simulink model "h_bridge_cascaded_five_level_inverter"  (R2022b)
settings: Solver=ode3  StartTime=0.0  StopTime=0.045  FixedStep=1e-6  RelTol=1e-3  EnableMultiTasking=on
undefined symbols (not defined in the file): fc, fr, Ma, ph
libraries: spsIGBTDiodeLib x328, simulink x164, spsDCVoltageSourceLib x82, spsCurrentMeasurementLib x41, spsSeriesRLCBranchLib x41, spsVoltageMeasurementLib x41, spspowerguiLib x1
(part 1 of 3)
settings Model: Creator=sruthi  LastModifiedBy=neotod
settings SolverCC: AlgebraicLoopSolver=TrustRegion  AutoInsertRateTranBlk=on
settings DataIOCC: LimitDataPoints=on  SaveFormat=Array  SignalLoggingSaveFormat=ModelDataLogs  ReturnWorkspaceOutputs=off
settings OptimizationCC: ExpressionDepthLimit=2147483647  LifeSpan=inf
settings DebuggingCC: UnderspecifiedInitializationDetection=Classic  MergeDetectMultiDrivingBlocksExec=none  SolverPrmCheckMsg=warning  FcnCallInpInsideContextMsg=warning  UnconnectedInputMsg=warning  UnconnectedOutputMsg=warning  UnconnectedLineMsg=warning  StateNameClashWarn=warning  SFUnexpectedBacktrackingDiag=warning  SFNoUnconditionalDefaultTransitionDiag=warning  SFExecutionAtInitializationDiag=none  SFMachineParentedDataDiag=warning  ArithmeticOperatorsInVariantConditions=warning
settings HardwareCC: ProdBitPerPointer=32  ProdBitPerSizeT=32  ProdBitPerPtrDiffT=32  ProdLargestAtomicFloat=None  ProdIntDivRoundTo=Undefined  ProdEndianess=Unspecified  ProdWordSize=32  ProdHWDeviceType=32-bit Generic
settings ModelReferenceCC: PropagateSignalLabelsOutOfModel=off
settings SFSimCC: SimUseLocalCustomCode=off  CustomCodeUndefinedFunction=UseInterfaceOnly
settings RTWCC: RTWUseLocalCustomCode=off
settings CodeAppCC: StateflowObjectComments=on
settings GRTTargetCC: TargetLangStandard=C89/C90 (ANSI)  CombineOutputUpdateFcns=off  GRTInterface=on
settings ConfigComp: CovMetricSettings=dw  CovSaveCumulativeToWorkspaceVar=on  CovSaveSingleToWorkspaceVar=on  CovExternalEMLEnable=off

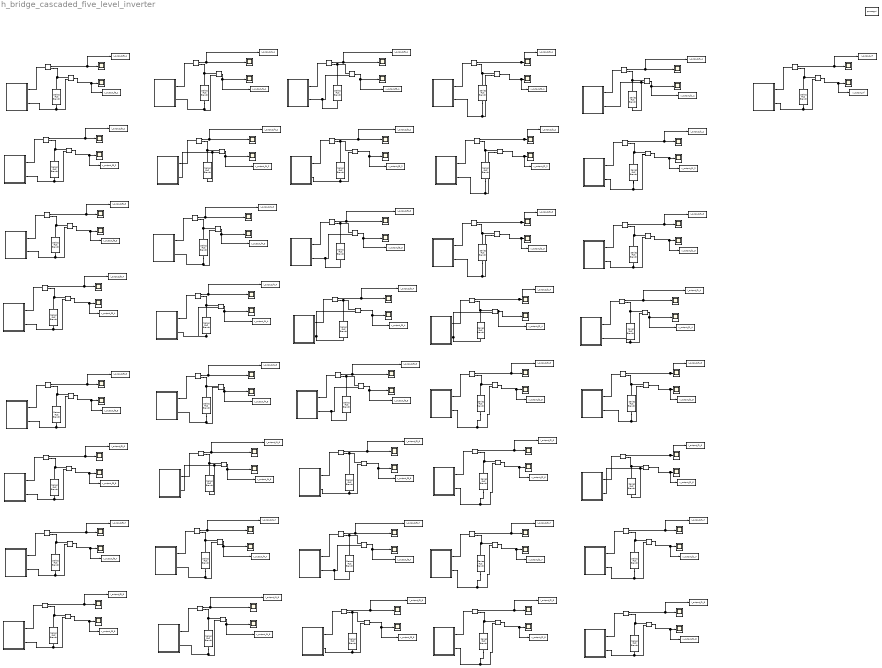
== system h_bridge_cascaded_five_level_inverter ==
  note: i_output_f6_5
  note: i_output_f3_6
  note: sim( '/path_to_simulinkmodel.slx' )
  note: currents
  note: voltages
  note: currents
  note: voltages
  note: currents
  note: voltages
  note: currents
  note: voltages
  note: CE short
  note: no fault
  note: collector open circuit
  note: gate signal removal
  note: voltages
  note: currents
  note: voltages
  note: currents
  note: voltages
  note: currents
  note: voltages
  note: voltages
  note: currents
  note: currents
  note: voltages
  note: voltages
  note: currents
  note: currents
  note: currents
  note: voltages
  note: emitter open circuit
  note: voltages
  note: currents
  note: currents
  note: voltages
  note: voltages
  note: currents
  note: voltages
  note: voltages
  note: currents
  note: currents
  note: currents
  note: voltages
  note: currents
  note: voltages
  note: voltages
  note: currents
  note: voltages
  note: currents
  note: voltages
  note: currents
  note: voltages
  note: currents
  note: voltages
  note: voltages
  note: currents
  note: voltages
  note: currents
  note: currents
  note: voltages
  note: currents
  note: voltages
  note: currents
  note: voltages
  note: currents
  note: currents
  note: voltages
  note: voltages
  note: voltages
  note: currents
  note: voltages
  note: currents
  note: currents
  note: voltages
  note: currents
  note: loose connection
  note: voltages
  note: currents
  note: voltages
  note: currents
  note: currents
  note: voltages
  note: voltages
  note: currents
  note: currents
  note: voltages
  note: voltages
  note: currents
  note: currents
  note: voltages
  Current Measurement{,1..3,5..34,42..48} (41 alike) : spsCurrentMeasurementLib/Current Measurement  PhasorSimulation=off  OutputType=Complex  PSBequivalent=0
  Phase A : Subsystem
  Phase A1 : Subsystem
  Phase A10 : Subsystem
  Phase A11 : Subsystem
  Phase A12 : Subsystem
  Phase A13 : Subsystem
  Phase A14 : Subsystem
  Phase A15 : Subsystem
  Phase A16 : Subsystem
  Phase A17 : Subsystem
  Phase A18 : Subsystem
  Phase A19 : Subsystem
  Phase A2 : Subsystem
  Phase A20 : Subsystem
  Phase A21 : Subsystem
  Phase A22 : Subsystem
  Phase A23 : Subsystem
  Phase A24 : Subsystem
  Phase A25 : Subsystem
  Phase A26 : Subsystem
  Phase A27 : Subsystem
  Phase A28 : Subsystem
  Phase A29 : Subsystem
  Phase A3 : Subsystem
  Phase A30 : Subsystem
  Phase A31 : Subsystem
  Phase A32 : Subsystem
  Phase A33 : Subsystem
  Phase A34 : Subsystem
  Phase A42 : Subsystem
  Phase A43 : Subsystem
  Phase A44 : Subsystem
  Phase A45 : Subsystem
  Phase A46 : Subsystem
  Phase A47 : Subsystem
  Phase A48 : Subsystem
  Phase A5 : Subsystem
  Phase A6 : Subsystem
  Phase A7 : Subsystem
  Phase A8 : Subsystem
  Phase A9 : Subsystem
  Scope{1..4,6..35,43..49} (41 alike) : Scope
  Series RLC Branch{,1..3,5..34,42..48} (41 alike) : spsSeriesRLCBranchLib/Series RLC Branch  LConnTagsString=__new0  RConnTagsString=__new0  BranchType=RL  Resistance=5  Inductance=5e-3  SetiL0=off  InitialCurrent=0  Capacitance=1e-6  Setx0=off  InitialVoltage=0  Measurements=None
  To Workspace : ToWorkspace  VariableName=v_output_nf  SaveFormat=Timeseries  SampleTime=-1
  To Workspace1 : ToWorkspace  VariableName=v_output_f1_1  SaveFormat=Timeseries  SampleTime=-1
  To Workspace10 : ToWorkspace  VariableName=v_output_f4_1  SaveFormat=Timeseries  SampleTime=-1
  To Workspace11 : ToWorkspace  VariableName=i_output_f4_1  SaveFormat=Timeseries  SampleTime=-1
  To Workspace12 : ToWorkspace  VariableName=v_output_f5_1  SaveFormat=Timeseries  SampleTime=-1
  To Workspace13 : ToWorkspace  VariableName=i_output_f5_1  SaveFormat=Timeseries  SampleTime=-1
  To Workspace14 : ToWorkspace  VariableName=v_output_f1_2  SaveFormat=Timeseries  SampleTime=-1
  To Workspace15 : ToWorkspace  VariableName=i_output_f1_2  SaveFormat=Timeseries  SampleTime=-1
  To Workspace16 : ToWorkspace  VariableName=v_output_f1_3  SaveFormat=Timeseries  SampleTime=-1
  To Workspace17 : ToWorkspace  VariableName=i_output_f1_3  SaveFormat=Timeseries  SampleTime=-1
  To Workspace18 : ToWorkspace  VariableName=v_output_f1_4  SaveFormat=Timeseries  SampleTime=-1
  To Workspace19 : ToWorkspace  VariableName=v_output_f1_5  SaveFormat=Timeseries  SampleTime=-1
  To Workspace2 : ToWorkspace  VariableName=i_output_f1_1  SaveFormat=Timeseries  SampleTime=-1
  To Workspace20 : ToWorkspace  VariableName=i_output_f1_5  SaveFormat=Timeseries  SampleTime=-1
  To Workspace21 : ToWorkspace  VariableName=v_output_f1_6  SaveFormat=Timeseries  SampleTime=-1
  To Workspace22 : ToWorkspace  VariableName=i_output_f1_6  SaveFormat=Timeseries  SampleTime=-1
  To Workspace23 : ToWorkspace  VariableName=i_output_f1_4  SaveFormat=Timeseries  SampleTime=-1
  To Workspace24 : ToWorkspace  VariableName=v_output_f1_7  SaveFormat=Timeseries  SampleTime=-1
  To Workspace25 : ToWorkspace  VariableName=i_output_f1_7  SaveFormat=Timeseries  SampleTime=-1
  To Workspace26 : ToWorkspace  VariableName=v_output_f1_8  SaveFormat=Timeseries  SampleTime=-1
  To Workspace27 : ToWorkspace  VariableName=i_output_f1_8  SaveFormat=Timeseries  SampleTime=-1
  To Workspace28 : ToWorkspace  VariableName=v_output_f2_2  SaveFormat=Timeseries  SampleTime=-1
  To Workspace29 : ToWorkspace  VariableName=i_output_f2_2  SaveFormat=Timeseries  SampleTime=-1
  To Workspace3 : ToWorkspace  VariableName=i_output_nf  SaveFormat=Timeseries  SampleTime=-1
  To Workspace30 : ToWorkspace  VariableName=v_output_f2_4  SaveFormat=Timeseries  SampleTime=-1
  To Workspace31 : ToWorkspace  VariableName=i_output_f2_4  SaveFormat=Timeseries  SampleTime=-1
  To Workspace32 : ToWorkspace  VariableName=v_output_f2_3  SaveFormat=Timeseries  SampleTime=-1
  To Workspace33 : ToWorkspace  VariableName=i_output_f2_3  SaveFormat=Timeseries  SampleTime=-1
  To Workspace34 : ToWorkspace  VariableName=v_output_f2_6  SaveFormat=Timeseries  SampleTime=-1
  To Workspace35 : ToWorkspace  VariableName=i_output_f2_6  SaveFormat=Timeseries  SampleTime=-1
  To Workspace36 : ToWorkspace  VariableName=v_output_f2_8  SaveFormat=Timeseries  SampleTime=-1
  To Workspace37 : ToWorkspace  VariableName=i_output_f2_8  SaveFormat=Timeseries  SampleTime=-1
  To Workspace38 : ToWorkspace  VariableName=v_output_f2_7  SaveFormat=Timeseries  SampleTime=-1
  To Workspace39 : ToWorkspace  VariableName=i_output_f2_7  SaveFormat=Timeseries  SampleTime=-1
  To Workspace4 : ToWorkspace  VariableName=v_output_f2_1  SaveFormat=Timeseries  SampleTime=-1
  To Workspace40 : ToWorkspace  VariableName=v_output_f2_5  SaveFormat=Timeseries  SampleTime=-1
  To Workspace41 : ToWorkspace  VariableName=i_output_f2_5  SaveFormat=Timeseries  SampleTime=-1
  To Workspace42 : ToWorkspace  VariableName=v_output_f3_2  SaveFormat=Timeseries  SampleTime=-1
  To Workspace43 : ToWorkspace  VariableName=i_output_f3_2  SaveFormat=Timeseries  SampleTime=-1
  To Workspace44 : ToWorkspace  VariableName=v_output_f3_4  SaveFormat=Timeseries  SampleTime=-1
  To Workspace45 : ToWorkspace  VariableName=i_output_f3_4  SaveFormat=Timeseries  SampleTime=-1
  To Workspace46 : ToWorkspace  VariableName=v_output_f3_3  SaveFormat=Timeseries  SampleTime=-1
  To Workspace47 : ToWorkspace  VariableName=i_output_f3_3  SaveFormat=Timeseries  SampleTime=-1
  To Workspace48 : ToWorkspace  VariableName=v_output_f3_6  SaveFormat=Timeseries  SampleTime=-1
  To Workspace49 : ToWorkspace  VariableName=i_output_f3_6  SaveFormat=Timeseries  SampleTime=-1
  To Workspace5 : ToWorkspace  VariableName=i_output_f2_1  SaveFormat=Timeseries  SampleTime=-1
  To Workspace50 : ToWorkspace  VariableName=v_output_f3_8  SaveFormat=Timeseries  SampleTime=-1
  To Workspace51 : ToWorkspace  VariableName=i_output_f3_8  SaveFormat=Timeseries  SampleTime=-1
  To Workspace52 : ToWorkspace  VariableName=v_output_f3_7  SaveFormat=Timeseries  SampleTime=-1
  To Workspace53 : ToWorkspace  VariableName=i_output_f3_7  SaveFormat=Timeseries  SampleTime=-1
  To Workspace54 : ToWorkspace  VariableName=v_output_f3_5  SaveFormat=Timeseries  SampleTime=-1
  To Workspace55 : ToWorkspace  VariableName=i_output_f3_5  SaveFormat=Timeseries  SampleTime=-1
  To Workspace56 : ToWorkspace  VariableName=v_output_f4_2  SaveFormat=Timeseries  SampleTime=-1
  To Workspace57 : ToWorkspace  VariableName=i_output_f4_2  SaveFormat=Timeseries  SampleTime=-1
  To Workspace58 : ToWorkspace  VariableName=v_output_f4_3  SaveFormat=Timeseries  SampleTime=-1
  To Workspace59 : ToWorkspace  VariableName=i_output_f4_3  SaveFormat=Timeseries  SampleTime=-1
  To Workspace6 : ToWorkspace  VariableName=v_output_f3_1  SaveFormat=Timeseries  SampleTime=-1
  To Workspace60 : ToWorkspace  VariableName=v_output_f4_4  SaveFormat=Timeseries  SampleTime=-1
  To Workspace61 : ToWorkspace  VariableName=i_output_f4_4  SaveFormat=Timeseries  SampleTime=-1
  To Workspace62 : ToWorkspace  VariableName=v_output_f4_5  SaveFormat=Timeseries  SampleTime=-1
  To Workspace63 : ToWorkspace  VariableName=i_output_f4_5  SaveFormat=Timeseries  SampleTime=-1
  To Workspace64 : ToWorkspace  VariableName=v_output_f4_6  SaveFormat=Timeseries  SampleTime=-1
  To Workspace65 : ToWorkspace  VariableName=i_output_f4_6  SaveFormat=Timeseries  SampleTime=-1
  To Workspace66 : ToWorkspace  VariableName=v_output_f4_7  SaveFormat=Timeseries  SampleTime=-1
  To Workspace67 : ToWorkspace  VariableName=i_output_f4_7  SaveFormat=Timeseries  SampleTime=-1
  To Workspace68 : ToWorkspace  VariableName=v_output_f4_8  SaveFormat=Timeseries  SampleTime=-1
  To Workspace69 : ToWorkspace  VariableName=i_output_f4_8  SaveFormat=Timeseries  SampleTime=-1
  To Workspace7 : ToWorkspace  VariableName=i_output_f3_1  SaveFormat=Timeseries  SampleTime=-1
  To Workspace84 : ToWorkspace  VariableName=v_output_f5_2  SaveFormat=Timeseries  SampleTime=-1
  To Workspace85 : ToWorkspace  VariableName=i_output_f5_2  SaveFormat=Timeseries  SampleTime=-1
  To Workspace86 : ToWorkspace  VariableName=v_output_f5_3  SaveFormat=Timeseries  SampleTime=-1
  To Workspace87 : ToWorkspace  VariableName=i_output_f5_3  SaveFormat=Timeseries  SampleTime=-1
  To Workspace88 : ToWorkspace  VariableName=v_output_f5_4  SaveFormat=Timeseries  SampleTime=-1
  To Workspace89 : ToWorkspace  VariableName=i_output_f5_4  SaveFormat=Timeseries  SampleTime=-1
  To Workspace90 : ToWorkspace  VariableName=v_output_f5_5  SaveFormat=Timeseries  SampleTime=-1
  To Workspace91 : ToWorkspace  VariableName=i_output_f5_5  SaveFormat=Timeseries  SampleTime=-1
  To Workspace92 : ToWorkspace  VariableName=v_output_f5_6  SaveFormat=Timeseries  SampleTime=-1
  To Workspace93 : ToWorkspace  VariableName=i_output_f5_6  SaveFormat=Timeseries  SampleTime=-1
  To Workspace94 : ToWorkspace  VariableName=v_output_f5_7  SaveFormat=Timeseries  SampleTime=-1
  To Workspace95 : ToWorkspace  VariableName=i_output_f5_7  SaveFormat=Timeseries  SampleTime=-1
  To Workspace96 : ToWorkspace  VariableName=v_output_f5_8  SaveFormat=Timeseries  SampleTime=-1
  To Workspace97 : ToWorkspace  VariableName=i_output_f5_8  SaveFormat=Timeseries  SampleTime=-1
  Voltage Measurement{,1..3,5..34,42..48} (41 alike) : spsVoltageMeasurementLib/Voltage Measurement  PhasorSimulation=off  OutputType=Complex  PSBequivalent=0
  current{,1..3,5..34,42..48} (41 alike) : Scope
  powergui : spspowerguiLib/powergui  Priority=1  SimulationMode=Discrete  SampleTime=100e-6  frequency=60  Iterations=50  frequencyindice=0  Pbase=100e6  ErrMax=1e-4  UnitsV=kV  UnitsW=MW  buscounter=0  FunctionMessages=off  echomessages=off  EnableUseOfTLC=off  CurrentSourceSwitches=off  DisableSnubberDevices=off  DisableRonSwitches=off  DisableVfSwitches=off  DisplayEquations=off  AutomaticDiscreteSolvers=off  SolverType=Tustin/Backward Euler (TBE)  Interpol=off  ExternalGateDelay=off  methode=off  Ts=100  x0status=blocks  SPID=off  SwTol=0  HookPort=off  NonlinearTolerance=1e-4  nMaxIteration=100  ContinueOnMaxIteration=off  RestoreLinks=warning  ResistiveCurrentMeasurement=off  Frange=[0:2:500]  Ylog=off  Xlog=on  ShowGrid=off  save=off  variable=ZData  structure=ScopeData  ZoomFFT=on  StartTime=0.0  cycles=1  DisplayStyle=1  fundamental=60  FreqAxis=off  MaxFrequency=1000  frequencyindicesteady=1  RmsSteady=1  display=off
  wires:
  Voltage Measurement/1 -> To Workspace/1, Scope1/1
  Current Measurement/1 -> To Workspace3/1, current/1
  Current Measurement1/1 -> To Workspace2/1, current1/1
  Voltage Measurement1/1 -> To Workspace1/1, Scope2/1
  Voltage Measurement3/1 -> To Workspace6/1, Scope4/1
  Current Measurement3/1 -> To Workspace7/1, current3/1
  Current Measurement5/1 -> To Workspace11/1, current5/1
  Voltage Measurement5/1 -> To Workspace10/1, Scope6/1
  Current Measurement7/1 -> To Workspace15/1, current7/1
  Voltage Measurement7/1 -> To Workspace14/1, Scope8/1
  Voltage Measurement8/1 -> To Workspace16/1, Scope9/1
  Current Measurement8/1 -> To Workspace17/1, current8/1
  Voltage Measurement11/1 -> To Workspace21/1, Scope12/1
  Voltage Measurement10/1 -> To Workspace19/1, Scope11/1
  Current Measurement11/1 -> To Workspace22/1, current11/1
  Current Measurement9/1 -> To Workspace23/1, current9/1
  Voltage Measurement9/1 -> To Workspace18/1, Scope10/1
  Current Measurement10/1 -> To Workspace20/1, current10/1
  Current Measurement13/1 -> To Workspace27/1, current13/1
  Voltage Measurement12/1 -> To Workspace24/1, Scope13/1
  Voltage Measurement13/1 -> To Workspace26/1, Scope14/1
  Current Measurement12/1 -> To Workspace25/1, current12/1
  Voltage Measurement2/1 -> To Workspace4/1, Scope3/1
  Current Measurement2/1 -> To Workspace5/1, current2/1
  Current Measurement14/1 -> To Workspace29/1, current14/1
  Voltage Measurement14/1 -> To Workspace28/1, Scope15/1
  Current Measurement15/1 -> To Workspace31/1, current15/1
  Voltage Measurement15/1 -> To Workspace30/1, Scope16/1
  Current Measurement16/1 -> To Workspace33/1, current16/1
  Voltage Measurement16/1 -> To Workspace32/1, Scope17/1
  Current Measurement17/1 -> To Workspace35/1, current17/1
  Voltage Measurement17/1 -> To Workspace34/1, Scope18/1
  Voltage Measurement19/1 -> To Workspace38/1, Scope20/1
  Voltage Measurement18/1 -> To Workspace36/1, Scope19/1
  Current Measurement18/1 -> To Workspace37/1, current18/1
  Current Measurement19/1 -> To Workspace39/1, current19/1
  Current Measurement20/1 -> To Workspace41/1, current20/1
  Voltage Measurement20/1 -> To Workspace40/1, Scope21/1
  Current Measurement21/1 -> To Workspace43/1, current21/1
  Voltage Measurement21/1 -> To Workspace42/1, Scope22/1
  Voltage Measurement22/1 -> To Workspace44/1, Scope23/1
  Current Measurement22/1 -> To Workspace45/1, current22/1
  Current Measurement23/1 -> To Workspace47/1, current23/1
  Voltage Measurement23/1 -> To Workspace46/1, Scope24/1
  Voltage Measurement24/1 -> To Workspace48/1, Scope25/1
  Current Measurement24/1 -> To Workspace49/1, current24/1
  Voltage Measurement27/1 -> To Workspace54/1, Scope28/1
  Current Measurement26/1 -> To Workspace53/1, current26/1
  Voltage Measurement26/1 -> To Workspace52/1, Scope27/1
  Current Measurement25/1 -> To Workspace51/1, current25/1
  Current Measurement27/1 -> To Workspace55/1, current27/1
  Voltage Measurement25/1 -> To Workspace50/1, Scope26/1
  Current Measurement28/1 -> To Workspace57/1, current28/1
  Voltage Measurement28/1 -> To Workspace56/1, Scope29/1
  Voltage Measurement29/1 -> To Workspace60/1, Scope30/1
  Current Measurement29/1 -> To Workspace61/1, current29/1
  Current Measurement30/1 -> To Workspace59/1, current30/1
  Voltage Measurement30/1 -> To Workspace58/1, Scope31/1
  Current Measurement33/1 -> To Workspace67/1, current33/1
  Current Measurement32/1 -> To Workspace69/1, current32/1
  Voltage Measurement33/1 -> To Workspace66/1, Scope34/1
  Voltage Measurement32/1 -> To Workspace68/1, Scope33/1
  Voltage Measurement31/1 -> To Workspace64/1, Scope32/1
  Current Measurement31/1 -> To Workspace65/1, current31/1
  Current Measurement34/1 -> To Workspace63/1, current34/1
  Voltage Measurement34/1 -> To Workspace62/1, Scope35/1
  Voltage Measurement6/1 -> To Workspace12/1, Scope7/1
  Current Measurement6/1 -> To Workspace13/1, current6/1
  Current Measurement42/1 -> To Workspace85/1, current42/1
  Voltage Measurement42/1 -> To Workspace84/1, Scope43/1
  Current Measurement44/1 -> To Workspace87/1, current44/1
  Voltage Measurement44/1 -> To Workspace86/1, Scope45/1
  Current Measurement43/1 -> To Workspace89/1, current43/1
  Voltage Measurement43/1 -> To Workspace88/1, Scope44/1
  Voltage Measurement47/1 -> To Workspace94/1, Scope48/1
  Voltage Measurement46/1 -> To Workspace96/1, Scope47/1
  Current Measurement48/1 -> To Workspace91/1, current48/1
  Current Measurement47/1 -> To Workspace95/1, current47/1
  Voltage Measurement48/1 -> To Workspace90/1, Scope49/1
  Current Measurement45/1 -> To Workspace93/1, current45/1
  Current Measurement46/1 -> To Workspace97/1, current46/1
  Voltage Measurement45/1 -> To Workspace92/1, Scope46/1
  connections:
  Voltage Measurement/LConn1 -- Series RLC Branch/LConn1 -- Current Measurement/RConn1
  Phase A/RConn1 -- Current Measurement/LConn1
  Phase A/RConn2 -- Series RLC Branch/RConn1 -- Voltage Measurement/LConn2
  Current Measurement1/RConn1 -- Series RLC Branch1/LConn1 -- Voltage Measurement1/LConn1
  Series RLC Branch1/RConn1 -- Phase A1/RConn2 -- Voltage Measurement1/LConn2
  Phase A1/RConn1 -- Current Measurement1/LConn1
  Phase A3/RConn2 -- Voltage Measurement3/LConn2 -- Series RLC Branch3/RConn1
  Current Measurement3/RConn1 -- Series RLC Branch3/LConn1 -- Voltage Measurement3/LConn1
  Phase A3/RConn1 -- Current Measurement3/LConn1
  Current Measurement5/RConn1 -- Series RLC Branch5/LConn1 -- Voltage Measurement5/LConn1
  Series RLC Branch5/RConn1 -- Phase A5/RConn2 -- Voltage Measurement5/LConn2
  Phase A5/RConn1 -- Current Measurement5/LConn1
  Voltage Measurement7/LConn2 -- Phase A7/RConn2 -- Series RLC Branch7/RConn1
  Current Measurement7/RConn1 -- Series RLC Branch7/LConn1 -- Voltage Measurement7/LConn1
  Phase A7/RConn1 -- Current Measurement7/LConn1
  Current Measurement8/RConn1 -- Series RLC Branch8/LConn1 -- Voltage Measurement8/LConn1
  Voltage Measurement8/LConn2 -- Phase A8/RConn2 -- Series RLC Branch8/RConn1
  Phase A8/RConn1 -- Current Measurement8/LConn1
  Current Measurement11/RConn1 -- Voltage Measurement11/LConn1 -- Series RLC Branch11/LConn1
  Current Measurement10/RConn1 -- Voltage Measurement10/LConn1 -- Series RLC Branch10/LConn1
  Voltage Measurement10/LConn2 -- Phase A10/RConn2 -- Series RLC Branch10/RConn1
  Current Measurement9/RConn1 -- Series RLC Branch9/LConn1 -- Voltage Measurement9/LConn1
  Series RLC Branch9/RConn1 -- Voltage Measurement9/LConn2 -- Phase A9/RConn2
  Voltage Measurement11/LConn2 -- Phase A11/RConn2 -- Series RLC Branch11/RConn1
  Phase A10/RConn1 -- Current Measurement10/LConn1
  Phase A11/RConn1 -- Current Measurement11/LConn1
  Phase A9/RConn1 -- Current Measurement9/LConn1
  Voltage Measurement13/LConn2 -- Phase A13/RConn2 -- Series RLC Branch13/RConn1
  Current Measurement12/RConn1 -- Series RLC Branch12/LConn1 -- Voltage Measurement12/LConn1
  Current Measurement13/RConn1 -- Series RLC Branch13/LConn1 -- Voltage Measurement13/LConn1
  Voltage Measurement12/LConn2 -- Phase A12/RConn2 -- Series RLC Branch12/RConn1
  Phase A13/RConn1 -- Current Measurement13/LConn1
  Phase A12/RConn1 -- Current Measurement12/LConn1
  Voltage Measurement2/LConn2 -- Phase A2/RConn2 -- Series RLC Branch2/RConn1
  Current Measurement2/RConn1 -- Voltage Measurement2/LConn1 -- Series RLC Branch2/LConn1
  Phase A2/RConn1 -- Current Measurement2/LConn1
  Current Measurement14/RConn1 -- Voltage Measurement14/LConn1 -- Series RLC Branch14/LConn1
  Voltage Measurement14/LConn2 -- Phase A14/RConn2 -- Series RLC Branch14/RConn1
  Phase A14/RConn1 -- Current Measurement14/LConn1
  Phase A15/RConn2 -- Series RLC Branch15/RConn1 -- Voltage Measurement15/LConn2
  Current Measurement15/RConn1 -- Voltage Measurement15/LConn1 -- Series RLC Branch15/LConn1
  Current Measurement16/RConn1 -- Voltage Measurement16/LConn1 -- Series RLC Branch16/LConn1
  Voltage Measurement16/LConn2 -- Phase A16/RConn2 -- Series RLC Branch16/RConn1
  Phase A15/RConn1 -- Current Measurement15/LConn1
  Phase A16/RConn1 -- Current Measurement16/LConn1
  Current Measurement18/RConn1 -- Series RLC Branch18/LConn1 -- Voltage Measurement18/LConn1
  Current Measurement19/RConn1 -- Series RLC Branch19/LConn1 -- Voltage Measurement19/LConn1
  Voltage Measurement17/LConn2 -- Phase A17/RConn2 -- Series RLC Branch17/RConn1
  Voltage Measurement18/LConn2 -- Phase A18/RConn2 -- Series RLC Branch18/RConn1
  Current Measurement17/RConn1 -- Series RLC Branch17/LConn1 -- Voltage Measurement17/LConn1
  Current Measurement20/RConn1 -- Series RLC Branch20/LConn1 -- Voltage Measurement20/LConn1
  Voltage Measurement20/LConn2 -- Phase A20/RConn2 -- Series RLC Branch20/RConn1
  Voltage Measurement19/LConn2 -- Phase A19/RConn2 -- Series RLC Branch19/RConn1
  Phase A19/RConn1 -- Current Measurement19/LConn1
  Phase A20/RConn1 -- Current Measurement20/LConn1
  Phase A18/RConn1 -- Current Measurement18/LConn1
  Phase A17/RConn1 -- Current Measurement17/LConn1
  Phase A21/RConn2 -- Voltage Measurement21/LConn2 -- Series RLC Branch21/RConn1
  Voltage Measurement21/LConn1 -- Current Measurement21/RConn1 -- Series RLC Branch21/LConn1
  Phase A21/RConn1 -- Current Measurement21/LConn1
  Phase A22/RConn2 -- Voltage Measurement22/LConn2 -- Series RLC Branch22/RConn1
  Voltage Measurement22/LConn1 -- Current Measurement22/RConn1 -- Series RLC Branch22/LConn1
  Series RLC Branch23/RConn1 -- Phase A23/RConn2 -- Voltage Measurement23/LConn2
  Voltage Measurement23/LConn1 -- Current Measurement23/RConn1 -- Series RLC Branch23/LConn1
  Phase A22/RConn1 -- Current Measurement22/LConn1
  Phase A23/RConn1 -- Current Measurement23/LConn1
  Voltage Measurement25/LConn1 -- Current Measurement25/RConn1 -- Series RLC Branch25/LConn1
  Phase A25/RConn2 -- Voltage Measurement25/LConn2 -- Series RLC Branch25/RConn1
  Phase A24/RConn2 -- Voltage Measurement24/LConn2 -- Series RLC Branch24/RConn1
  Series RLC Branch26/RConn1 -- Phase A26/RConn2 -- Voltage Measurement26/LConn2
  Voltage Measurement24/LConn1 -- Current Measurement24/RConn1 -- Series RLC Branch24/LConn1
  Voltage Measurement26/LConn1 -- Current Measurement26/RConn1 -- Series RLC Branch26/LConn1
  Series RLC Branch27/RConn1 -- Phase A27/RConn2 -- Voltage Measurement27/LConn2
  Voltage Measurement27/LConn1 -- Current Measurement27/RConn1 -- Series RLC Branch27/LConn1
  Phase A27/RConn1 -- Current Measurement27/LConn1
  Phase A26/RConn1 -- Current Measurement26/LConn1
  Phase A25/RConn1 -- Current Measurement25/LConn1
  Phase A24/RConn1 -- Current Measurement24/LConn1
  Current Measurement28/RConn1 -- Series RLC Branch28/LConn1 -- Voltage Measurement28/LConn1
  Series RLC Branch28/RConn1 -- Voltage Measurement28/LConn2 -- Phase A28/RConn2
  Phase A28/RConn1 -- Current Measurement28/LConn1
  Series RLC Branch29/RConn1 -- Phase A29/RConn2 -- Voltage Measurement29/LConn2
  Current Measurement30/RConn1 -- Series RLC Branch30/LConn1 -- Voltage Measurement30/LConn1
  Current Measurement29/RConn1 -- Series RLC Branch29/LConn1 -- Voltage Measurement29/LConn1
  Series RLC Branch30/RConn1 -- Phase A30/RConn2 -- Voltage Measurement30/LConn2
  Phase A30/RConn1 -- Current Measurement30/LConn1
  Phase A29/RConn1 -- Current Measurement29/LConn1
  Current Measurement32/RConn1 -- Series RLC Branch32/LConn1 -- Voltage Measurement32/LConn1
  Series RLC Branch32/RConn1 -- Phase A32/RConn2 -- Voltage Measurement32/LConn2
  Series RLC Branch33/RConn1 -- Phase A33/RConn2 -- Voltage Measurement33/LConn2
  Current Measurement33/RConn1 -- Series RLC Branch33/LConn1 -- Voltage Measurement33/LConn1
  Phase A31/RConn2 -- Series RLC Branch31/RConn1 -- Voltage Measurement31/LConn2
  Current Measurement34/RConn1 -- Series RLC Branch34/LConn1 -- Voltage Measurement34/LConn1
  Current Measurement31/RConn1 -- Series RLC Branch31/LConn1 -- Voltage Measurement31/LConn1
  Series RLC Branch34/RConn1 -- Phase A34/RConn2 -- Voltage Measurement34/LConn2
  Phase A34/RConn1 -- Current Measurement34/LConn1
  Phase A31/RConn1 -- Current Measurement31/LConn1
  Phase A33/RConn1 -- Current Measurement33/LConn1
  Phase A32/RConn1 -- Current Measurement32/LConn1
  Current Measurement6/RConn1 -- Series RLC Branch6/LConn1 -- Voltage Measurement6/LConn1
  Voltage Measurement6/LConn2 -- Phase A6/RConn2 -- Series RLC Branch6/RConn1
  Phase A6/RConn1 -- Current Measurement6/LConn1
  Voltage Measurement42/LConn2 -- Phase A42/RConn2 -- Series RLC Branch42/RConn1
  Current Measurement42/RConn1 -- Series RLC Branch42/LConn1 -- Voltage Measurement42/LConn1
  Phase A42/RConn1 -- Current Measurement42/LConn1
  Voltage Measurement43/LConn2 -- Phase A43/RConn2 -- Series RLC Branch43/RConn1
  Current Measurement43/RConn1 -- Series RLC Branch43/LConn1 -- Voltage Measurement43/LConn1
  Voltage Measurement44/LConn2 -- Phase A44/RConn2 -- Series RLC Branch44/RConn1
  Current Measurement44/RConn1 -- Series RLC Branch44/LConn1 -- Voltage Measurement44/LConn1
  Phase A44/RConn1 -- Current Measurement44/LConn1
  Phase A43/RConn1 -- Current Measurement43/LConn1
  Voltage Measurement46/LConn2 -- Phase A46/RConn2 -- Series RLC Branch46/RConn1
  Voltage Measurement45/LConn2 -- Phase A45/RConn2 -- Series RLC Branch45/RConn1
  Current Measurement45/RConn1 -- Series RLC Branch45/LConn1 -- Voltage Measurement45/LConn1
  Voltage Measurement47/LConn2 -- Phase A47/RConn2 -- Series RLC Branch47/RConn1
  Current Measurement47/RConn1 -- Series RLC Branch47/LConn1 -- Voltage Measurement47/LConn1
  Voltage Measurement48/LConn2 -- Phase A48/RConn2 -- Series RLC Branch48/RConn1
  Current Measurement48/RConn1 -- Series RLC Branch48/LConn1 -- Voltage Measurement48/LConn1
  Current Measurement46/RConn1 -- Series RLC Branch46/LConn1 -- Voltage Measurement46/LConn1
  Phase A47/RConn1 -- Current Measurement47/LConn1
  Phase A46/RConn1 -- Current Measurement46/LConn1
  Phase A45/RConn1 -- Current Measurement45/LConn1
  Phase A48/RConn1 -- Current Measurement48/LConn1

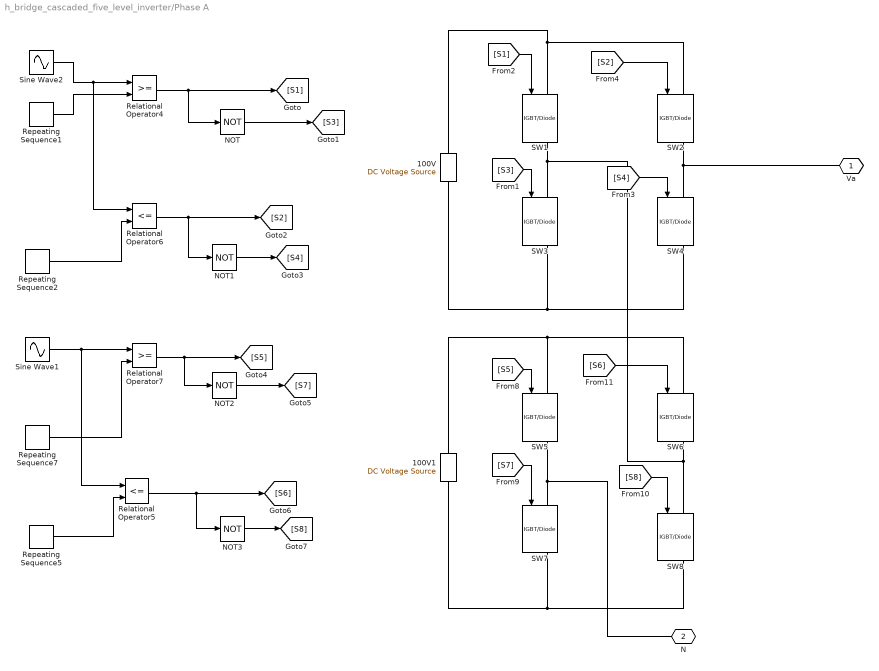
== system h_bridge_cascaded_five_level_inverter/Phase A ==
  100V : spsDCVoltageSourceLib/DC Voltage Source  Amplitude=100  Measurements=None
  100V1 : spsDCVoltageSourceLib/DC Voltage Source  Amplitude=100  Measurements=None
  NOT{,1..3} (4 alike) : Logic  Operator=NOT  AllPortsSameDT=off  OutDataTypeStr=boolean
  Relational Operator4 : RelationalOperator  OutDataTypeStr=boolean  InputSameDT=off
  Relational Operator5 : RelationalOperator  Operator=<=  OutDataTypeStr=boolean  InputSameDT=off
  Relational Operator6 : RelationalOperator  Operator=<=  OutDataTypeStr=boolean  InputSameDT=off
  Relational Operator7 : RelationalOperator  OutDataTypeStr=boolean  InputSameDT=off
  Repeating Sequence1 : simulink/Sources/Repeating Sequence  rep_seq_t=[0 0.00025 0.0005 0.00075 0.001]*(1/fr)*(1/fc)*(1/2)  rep_seq_y="[0 1 0 -1 0  ]"
  Repeating Sequence2 : simulink/Sources/Repeating Sequence  rep_seq_t=[0 0.00025 0.0005 0.00075 0.001]*(1/fr)*(1/fc)*(1/2)  rep_seq_y=[ 0 -1 0 1 0 ]
  Repeating Sequence5 : simulink/Sources/Repeating Sequence  rep_seq_t=[0 0.00025 0.0005 0.00075 0.001]*(1/fr)*(1/fc)*(1/2)  rep_seq_y=[1 0 -1 0 1]
  Repeating Sequence7 : simulink/Sources/Repeating Sequence  rep_seq_t=[0 0.00025 0.0005 0.00075 0.001]*(1/fr)*(1/fc)*(1/2)  rep_seq_y=[-1 0 1 0 -1]
  SW{1..8} (8 alike) : spsIGBTDiodeLib/IGBT//Diode  Ron=1e-3  Rs=1e5  Cs=inf  Measurements=on
  Sine Wave1 : Sin  Amplitude=Ma  Frequency=2*pi*fr  Phase=ph  SampleTime=0
  Sine Wave2 : Sin  Amplitude=Ma  Frequency=2*pi*fr  Phase=ph  SampleTime=0
  Va : PMIOPort  Tag=PMCPort  Side=Right
  N : PMIOPort  Tag=PMCPort  Port=2  Side=Right
  wires:
  Sine Wave2/1 -> Relational Operator4/1, Relational Operator6/1
  Repeating Sequence1/1 -> Relational Operator4/2
  Repeating Sequence2/1 -> Relational Operator6/2
  Relational Operator4/1 -> NOT/1, [S1]
  NOT/1 -> [S3]
  NOT1/1 -> [S4]
  Relational Operator6/1 -> [S2], NOT1/1
  Repeating Sequence7/1 -> Relational Operator7/2
  Repeating Sequence5/1 -> Relational Operator5/2
  Sine Wave1/1 -> Relational Operator7/1, Relational Operator5/1
  Relational Operator5/1 -> [S6], NOT3/1
  Relational Operator7/1 -> [S5], NOT2/1
  NOT2/1 -> [S7]
  NOT3/1 -> [S8]
  [S3] -> SW3/1
  [S4] -> SW4/1
  [S6] -> SW6/1
  [S5] -> SW5/1
  [S7] -> SW7/1
  [S8] -> SW8/1
  [S1] -> SW1/1
  [S2] -> SW2/1
  connections:
  Va/RConn1 -- SW2/RConn1 -- SW4/LConn1
  SW4/RConn1 -- 100V/LConn1 -- SW3/RConn1
  SW8/RConn1 -- 100V1/LConn1 -- SW7/RConn1
  SW1/RConn1 -- SW3/LConn1 -- SW6/RConn1 -- SW8/LConn1
  SW5/LConn1 -- 100V1/RConn1 -- SW6/LConn1
  N/RConn1 -- SW5/RConn1 -- SW7/LConn1
  100V/RConn1 -- SW2/LConn1 -- SW1/LConn1

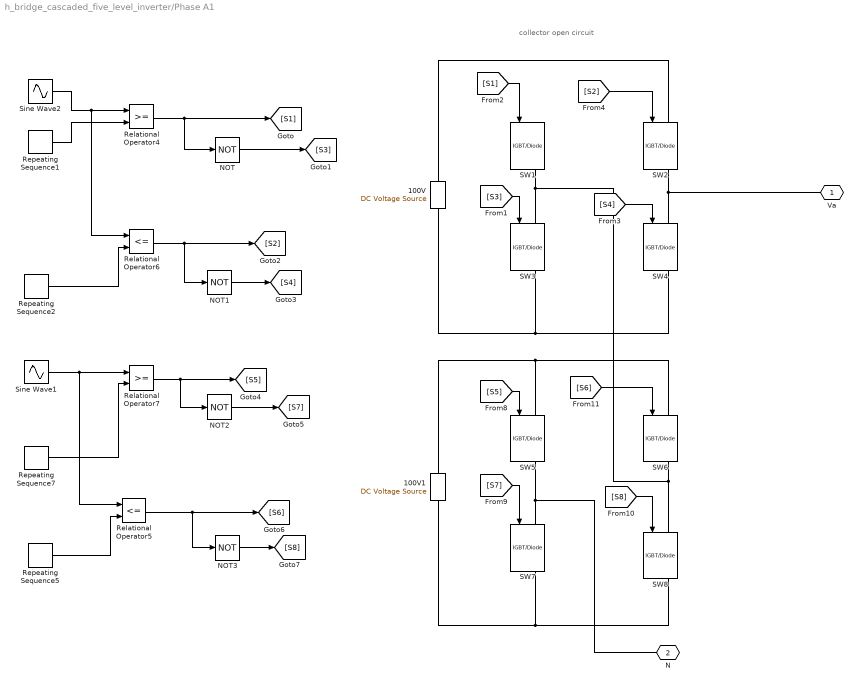
== system h_bridge_cascaded_five_level_inverter/Phase A1 ==
  note: collector open circuit
  100V : spsDCVoltageSourceLib/DC Voltage Source  Amplitude=100  Measurements=None
  100V1 : spsDCVoltageSourceLib/DC Voltage Source  Amplitude=100  Measurements=None
  NOT{,1..3} (4 alike) : Logic  Operator=NOT  AllPortsSameDT=off  OutDataTypeStr=boolean
  Relational Operator4 : RelationalOperator  OutDataTypeStr=boolean  InputSameDT=off
  Relational Operator5 : RelationalOperator  Operator=<=  OutDataTypeStr=boolean  InputSameDT=off
  Relational Operator6 : RelationalOperator  Operator=<=  OutDataTypeStr=boolean  InputSameDT=off
  Relational Operator7 : RelationalOperator  OutDataTypeStr=boolean  InputSameDT=off
  Repeating Sequence1 : simulink/Sources/Repeating Sequence  rep_seq_t=[0 0.00025 0.0005 0.00075 0.001]*(1/fr)*(1/fc)*(1/2)  rep_seq_y="[0 1 0 -1 0  ]"
  Repeating Sequence2 : simulink/Sources/Repeating Sequence  rep_seq_t=[0 0.00025 0.0005 0.00075 0.001]*(1/fr)*(1/fc)*(1/2)  rep_seq_y=[ 0 -1 0 1 0 ]
  Repeating Sequence5 : simulink/Sources/Repeating Sequence  rep_seq_t=[0 0.00025 0.0005 0.00075 0.001]*(1/fr)*(1/fc)*(1/2)  rep_seq_y=[1 0 -1 0 1]
  Repeating Sequence7 : simulink/Sources/Repeating Sequence  rep_seq_t=[0 0.00025 0.0005 0.00075 0.001]*(1/fr)*(1/fc)*(1/2)  rep_seq_y=[-1 0 1 0 -1]
  SW{1..8} (8 alike) : spsIGBTDiodeLib/IGBT//Diode  Ron=1e-3  Rs=1e5  Cs=inf  Measurements=on
  Sine Wave1 : Sin  Amplitude=Ma  Frequency=2*pi*fr  Phase=ph  SampleTime=0
  Sine Wave2 : Sin  Amplitude=Ma  Frequency=2*pi*fr  Phase=ph  SampleTime=0
  Va : PMIOPort  Tag=PMCPort  Side=Right
  N : PMIOPort  Tag=PMCPort  Port=2  Side=Right
  wires:
  Sine Wave2/1 -> Relational Operator4/1, Relational Operator6/1
  Repeating Sequence1/1 -> Relational Operator4/2
  Repeating Sequence2/1 -> Relational Operator6/2
  Relational Operator4/1 -> NOT/1, [S1]
  NOT/1 -> [S3]
  NOT1/1 -> [S4]
  Relational Operator6/1 -> [S2], NOT1/1
  Repeating Sequence7/1 -> Relational Operator7/2
  Repeating Sequence5/1 -> Relational Operator5/2
  Sine Wave1/1 -> Relational Operator7/1, Relational Operator5/1
  Relational Operator5/1 -> [S6], NOT3/1
  Relational Operator7/1 -> [S5], NOT2/1
  NOT2/1 -> [S7]
  NOT3/1 -> [S8]
  [S3] -> SW3/1
  [S4] -> SW4/1
  [S6] -> SW6/1
  [S5] -> SW5/1
  [S7] -> SW7/1
  [S8] -> SW8/1
  [S1] -> SW1/1
  [S2] -> SW2/1
  connections:
  Va/RConn1 -- SW2/RConn1 -- SW4/LConn1
  SW4/RConn1 -- 100V/LConn1 -- SW3/RConn1
  SW8/RConn1 -- 100V1/LConn1 -- SW7/RConn1
  SW1/RConn1 -- SW3/LConn1 -- SW6/RConn1 -- SW8/LConn1
  SW5/LConn1 -- 100V1/RConn1 -- SW6/LConn1
  N/RConn1 -- SW5/RConn1 -- SW7/LConn1
  SW2/LConn1 -- 100V/RConn1

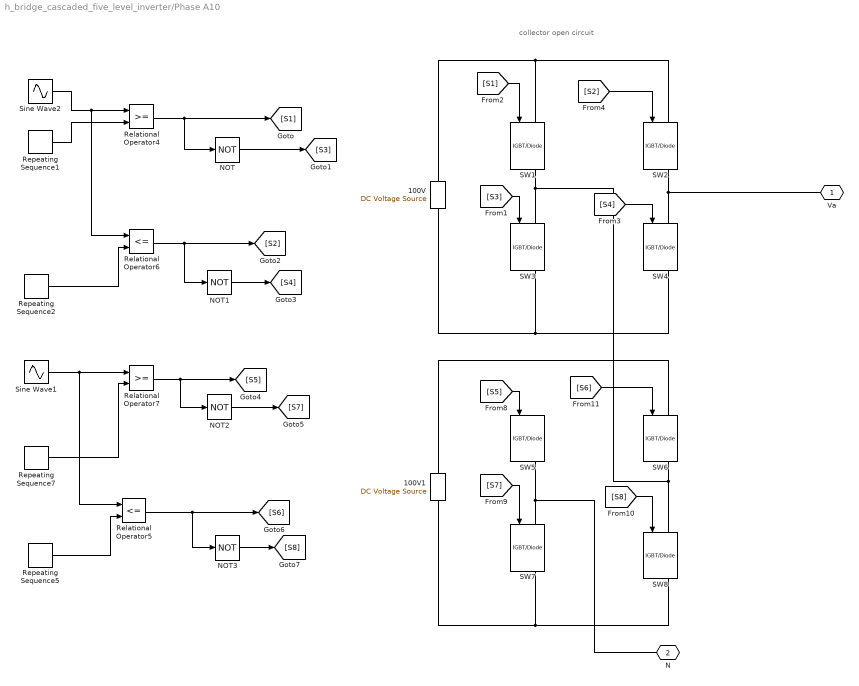
== system h_bridge_cascaded_five_level_inverter/Phase A10 ==
  note: collector open circuit
  100V : spsDCVoltageSourceLib/DC Voltage Source  Amplitude=100  Measurements=None
  100V1 : spsDCVoltageSourceLib/DC Voltage Source  Amplitude=100  Measurements=None
  NOT{,1..3} (4 alike) : Logic  Operator=NOT  AllPortsSameDT=off  OutDataTypeStr=boolean
  Relational Operator4 : RelationalOperator  OutDataTypeStr=boolean  InputSameDT=off
  Relational Operator5 : RelationalOperator  Operator=<=  OutDataTypeStr=boolean  InputSameDT=off
  Relational Operator6 : RelationalOperator  Operator=<=  OutDataTypeStr=boolean  InputSameDT=off
  Relational Operator7 : RelationalOperator  OutDataTypeStr=boolean  InputSameDT=off
  Repeating Sequence1 : simulink/Sources/Repeating Sequence  rep_seq_t=[0 0.00025 0.0005 0.00075 0.001]*(1/fr)*(1/fc)*(1/2)  rep_seq_y="[0 1 0 -1 0  ]"
  Repeating Sequence2 : simulink/Sources/Repeating Sequence  rep_seq_t=[0 0.00025 0.0005 0.00075 0.001]*(1/fr)*(1/fc)*(1/2)  rep_seq_y=[ 0 -1 0 1 0 ]
  Repeating Sequence5 : simulink/Sources/Repeating Sequence  rep_seq_t=[0 0.00025 0.0005 0.00075 0.001]*(1/fr)*(1/fc)*(1/2)  rep_seq_y=[1 0 -1 0 1]
  Repeating Sequence7 : simulink/Sources/Repeating Sequence  rep_seq_t=[0 0.00025 0.0005 0.00075 0.001]*(1/fr)*(1/fc)*(1/2)  rep_seq_y=[-1 0 1 0 -1]
  SW{1..8} (8 alike) : spsIGBTDiodeLib/IGBT//Diode  Ron=1e-3  Rs=1e5  Cs=inf  Measurements=on
  Sine Wave1 : Sin  Amplitude=Ma  Frequency=2*pi*fr  Phase=ph  SampleTime=0
  Sine Wave2 : Sin  Amplitude=Ma  Frequency=2*pi*fr  Phase=ph  SampleTime=0
  Va : PMIOPort  Tag=PMCPort  Side=Right
  N : PMIOPort  Tag=PMCPort  Port=2  Side=Right
  wires:
  Sine Wave2/1 -> Relational Operator4/1, Relational Operator6/1
  Repeating Sequence1/1 -> Relational Operator4/2
  Repeating Sequence2/1 -> Relational Operator6/2
  Relational Operator4/1 -> NOT/1, [S1]
  NOT/1 -> [S3]
  NOT1/1 -> [S4]
  Relational Operator6/1 -> [S2], NOT1/1
  Repeating Sequence7/1 -> Relational Operator7/2
  Repeating Sequence5/1 -> Relational Operator5/2
  Sine Wave1/1 -> Relational Operator7/1, Relational Operator5/1
  Relational Operator5/1 -> [S6], NOT3/1
  Relational Operator7/1 -> [S5], NOT2/1
  NOT2/1 -> [S7]
  NOT3/1 -> [S8]
  [S3] -> SW3/1
  [S4] -> SW4/1
  [S6] -> SW6/1
  [S5] -> SW5/1
  [S7] -> SW7/1
  [S8] -> SW8/1
  [S1] -> SW1/1
  [S2] -> SW2/1
  connections:
  Va/RConn1 -- SW2/RConn1 -- SW4/LConn1
  SW4/RConn1 -- 100V/LConn1 -- SW3/RConn1
  SW8/RConn1 -- 100V1/LConn1 -- SW7/RConn1
  SW1/RConn1 -- SW6/RConn1 -- SW8/LConn1 -- SW3/LConn1
  SW6/LConn1 -- 100V1/RConn1
  N/RConn1 -- SW5/RConn1 -- SW7/LConn1
  100V/RConn1 -- SW1/LConn1 -- SW2/LConn1

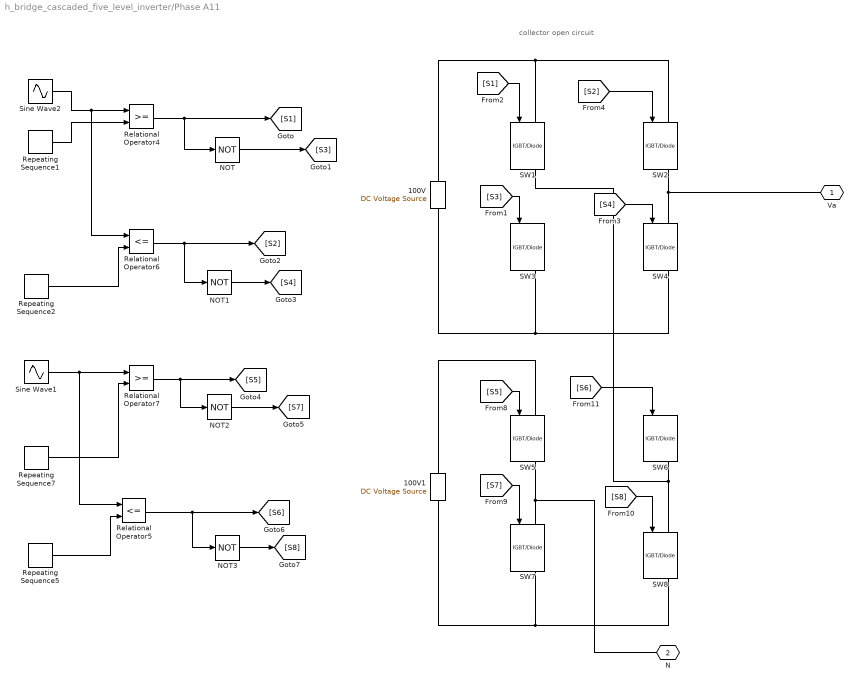
== system h_bridge_cascaded_five_level_inverter/Phase A11 ==
  note: collector open circuit
  100V : spsDCVoltageSourceLib/DC Voltage Source  Amplitude=100  Measurements=None
  100V1 : spsDCVoltageSourceLib/DC Voltage Source  Amplitude=100  Measurements=None
  NOT{,1..3} (4 alike) : Logic  Operator=NOT  AllPortsSameDT=off  OutDataTypeStr=boolean
  Relational Operator4 : RelationalOperator  OutDataTypeStr=boolean  InputSameDT=off
  Relational Operator5 : RelationalOperator  Operator=<=  OutDataTypeStr=boolean  InputSameDT=off
  Relational Operator6 : RelationalOperator  Operator=<=  OutDataTypeStr=boolean  InputSameDT=off
  Relational Operator7 : RelationalOperator  OutDataTypeStr=boolean  InputSameDT=off
  Repeating Sequence1 : simulink/Sources/Repeating Sequence  rep_seq_t=[0 0.00025 0.0005 0.00075 0.001]*(1/fr)*(1/fc)*(1/2)  rep_seq_y="[0 1 0 -1 0  ]"
  Repeating Sequence2 : simulink/Sources/Repeating Sequence  rep_seq_t=[0 0.00025 0.0005 0.00075 0.001]*(1/fr)*(1/fc)*(1/2)  rep_seq_y=[ 0 -1 0 1 0 ]
  Repeating Sequence5 : simulink/Sources/Repeating Sequence  rep_seq_t=[0 0.00025 0.0005 0.00075 0.001]*(1/fr)*(1/fc)*(1/2)  rep_seq_y=[1 0 -1 0 1]
  Repeating Sequence7 : simulink/Sources/Repeating Sequence  rep_seq_t=[0 0.00025 0.0005 0.00075 0.001]*(1/fr)*(1/fc)*(1/2)  rep_seq_y=[-1 0 1 0 -1]
  SW{1..8} (8 alike) : spsIGBTDiodeLib/IGBT//Diode  Ron=1e-3  Rs=1e5  Cs=inf  Measurements=on
  Sine Wave1 : Sin  Amplitude=Ma  Frequency=2*pi*fr  Phase=ph  SampleTime=0
  Sine Wave2 : Sin  Amplitude=Ma  Frequency=2*pi*fr  Phase=ph  SampleTime=0
  Va : PMIOPort  Tag=PMCPort  Side=Right
  N : PMIOPort  Tag=PMCPort  Port=2  Side=Right
  wires:
  Sine Wave2/1 -> Relational Operator4/1, Relational Operator6/1
  Repeating Sequence1/1 -> Relational Operator4/2
  Repeating Sequence2/1 -> Relational Operator6/2
  Relational Operator4/1 -> NOT/1, [S1]
  NOT/1 -> [S3]
  NOT1/1 -> [S4]
  Relational Operator6/1 -> [S2], NOT1/1
  Repeating Sequence7/1 -> Relational Operator7/2
  Repeating Sequence5/1 -> Relational Operator5/2
  Sine Wave1/1 -> Relational Operator7/1, Relational Operator5/1
  Relational Operator5/1 -> [S6], NOT3/1
  Relational Operator7/1 -> [S5], NOT2/1
  NOT2/1 -> [S7]
  NOT3/1 -> [S8]
  [S3] -> SW3/1
  [S4] -> SW4/1
  [S6] -> SW6/1
  [S5] -> SW5/1
  [S7] -> SW7/1
  [S8] -> SW8/1
  [S1] -> SW1/1
  [S2] -> SW2/1
  connections:
  Va/RConn1 -- SW2/RConn1 -- SW4/LConn1
  SW4/RConn1 -- 100V/LConn1 -- SW3/RConn1
  SW8/RConn1 -- 100V1/LConn1 -- SW7/RConn1
  SW6/RConn1 -- SW8/LConn1 -- SW1/RConn1
  100V1/RConn1 -- SW5/LConn1
  N/RConn1 -- SW5/RConn1 -- SW7/LConn1
  100V/RConn1 -- SW1/LConn1 -- SW2/LConn1

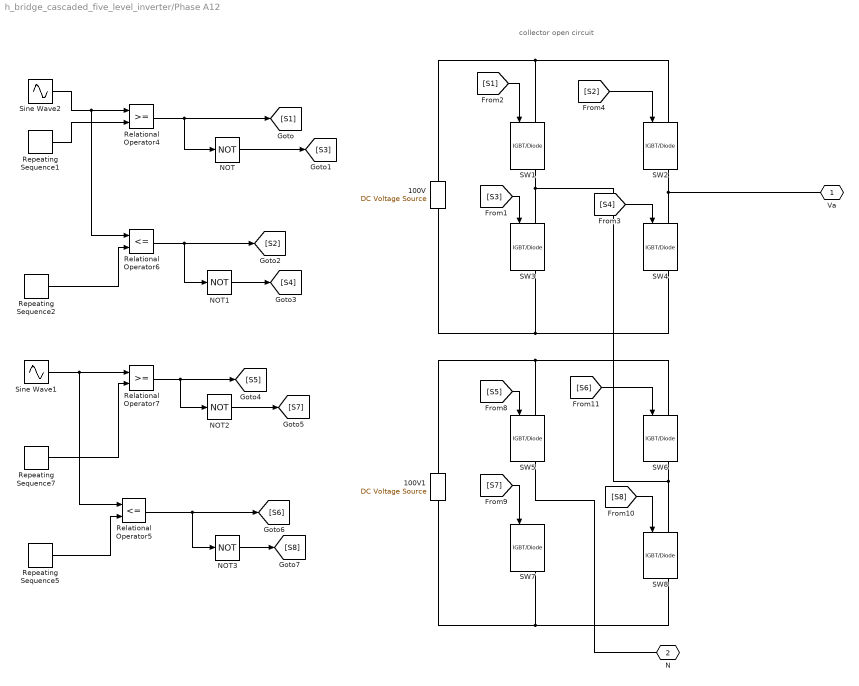
== system h_bridge_cascaded_five_level_inverter/Phase A12 ==
  note: collector open circuit
  100V : spsDCVoltageSourceLib/DC Voltage Source  Amplitude=100  Measurements=None
  100V1 : spsDCVoltageSourceLib/DC Voltage Source  Amplitude=100  Measurements=None
  NOT{,1..3} (4 alike) : Logic  Operator=NOT  AllPortsSameDT=off  OutDataTypeStr=boolean
  Relational Operator4 : RelationalOperator  OutDataTypeStr=boolean  InputSameDT=off
  Relational Operator5 : RelationalOperator  Operator=<=  OutDataTypeStr=boolean  InputSameDT=off
  Relational Operator6 : RelationalOperator  Operator=<=  OutDataTypeStr=boolean  InputSameDT=off
  Relational Operator7 : RelationalOperator  OutDataTypeStr=boolean  InputSameDT=off
  Repeating Sequence1 : simulink/Sources/Repeating Sequence  rep_seq_t=[0 0.00025 0.0005 0.00075 0.001]*(1/fr)*(1/fc)*(1/2)  rep_seq_y="[0 1 0 -1 0  ]"
  Repeating Sequence2 : simulink/Sources/Repeating Sequence  rep_seq_t=[0 0.00025 0.0005 0.00075 0.001]*(1/fr)*(1/fc)*(1/2)  rep_seq_y=[ 0 -1 0 1 0 ]
  Repeating Sequence5 : simulink/Sources/Repeating Sequence  rep_seq_t=[0 0.00025 0.0005 0.00075 0.001]*(1/fr)*(1/fc)*(1/2)  rep_seq_y=[1 0 -1 0 1]
  Repeating Sequence7 : simulink/Sources/Repeating Sequence  rep_seq_t=[0 0.00025 0.0005 0.00075 0.001]*(1/fr)*(1/fc)*(1/2)  rep_seq_y=[-1 0 1 0 -1]
  SW{1..8} (8 alike) : spsIGBTDiodeLib/IGBT//Diode  Ron=1e-3  Rs=1e5  Cs=inf  Measurements=on
  Sine Wave1 : Sin  Amplitude=Ma  Frequency=2*pi*fr  Phase=ph  SampleTime=0
  Sine Wave2 : Sin  Amplitude=Ma  Frequency=2*pi*fr  Phase=ph  SampleTime=0
  Va : PMIOPort  Tag=PMCPort  Side=Right
  N : PMIOPort  Tag=PMCPort  Port=2  Side=Right
  wires:
  Sine Wave2/1 -> Relational Operator4/1, Relational Operator6/1
  Repeating Sequence1/1 -> Relational Operator4/2
  Repeating Sequence2/1 -> Relational Operator6/2
  Relational Operator4/1 -> NOT/1, [S1]
  NOT/1 -> [S3]
  NOT1/1 -> [S4]
  Relational Operator6/1 -> [S2], NOT1/1
  Repeating Sequence7/1 -> Relational Operator7/2
  Repeating Sequence5/1 -> Relational Operator5/2
  Sine Wave1/1 -> Relational Operator7/1, Relational Operator5/1
  Relational Operator5/1 -> [S6], NOT3/1
  Relational Operator7/1 -> [S5], NOT2/1
  NOT2/1 -> [S7]
  NOT3/1 -> [S8]
  [S3] -> SW3/1
  [S4] -> SW4/1
  [S6] -> SW6/1
  [S5] -> SW5/1
  [S7] -> SW7/1
  [S8] -> SW8/1
  [S1] -> SW1/1
  [S2] -> SW2/1
  connections:
  Va/RConn1 -- SW2/RConn1 -- SW4/LConn1
  SW4/RConn1 -- 100V/LConn1 -- SW3/RConn1
  SW8/RConn1 -- 100V1/LConn1 -- SW7/RConn1
  SW1/RConn1 -- SW6/RConn1 -- SW8/LConn1 -- SW3/LConn1
  SW6/LConn1 -- SW5/LConn1 -- 100V1/RConn1
  SW5/RConn1 -- N/RConn1
  100V/RConn1 -- SW1/LConn1 -- SW2/LConn1

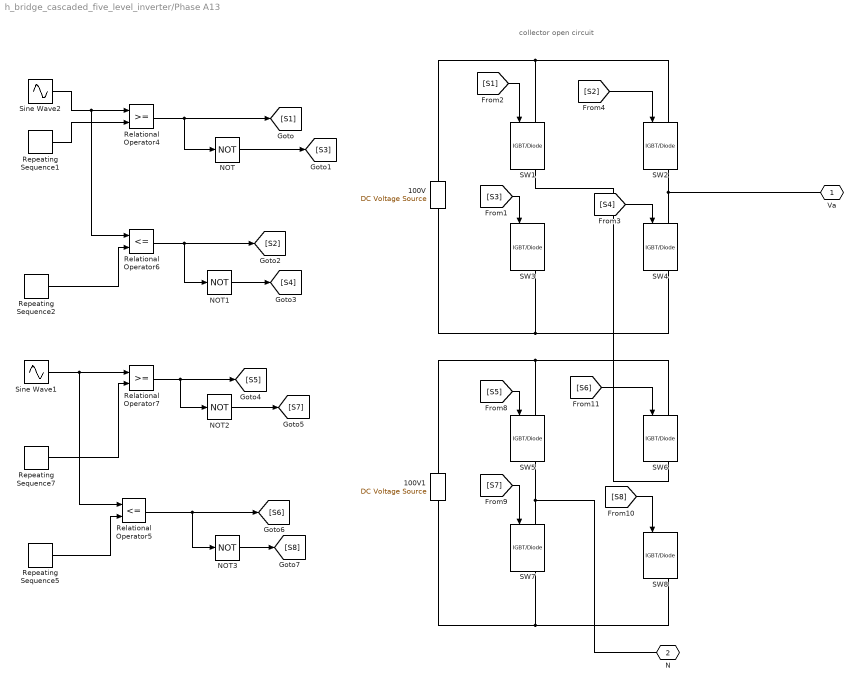
== system h_bridge_cascaded_five_level_inverter/Phase A13 ==
  note: collector open circuit
  100V : spsDCVoltageSourceLib/DC Voltage Source  Amplitude=100  Measurements=None
  100V1 : spsDCVoltageSourceLib/DC Voltage Source  Amplitude=100  Measurements=None
  NOT{,1..3} (4 alike) : Logic  Operator=NOT  AllPortsSameDT=off  OutDataTypeStr=boolean
  Relational Operator4 : RelationalOperator  OutDataTypeStr=boolean  InputSameDT=off
  Relational Operator5 : RelationalOperator  Operator=<=  OutDataTypeStr=boolean  InputSameDT=off
  Relational Operator6 : RelationalOperator  Operator=<=  OutDataTypeStr=boolean  InputSameDT=off
  Relational Operator7 : RelationalOperator  OutDataTypeStr=boolean  InputSameDT=off
  Repeating Sequence1 : simulink/Sources/Repeating Sequence  rep_seq_t=[0 0.00025 0.0005 0.00075 0.001]*(1/fr)*(1/fc)*(1/2)  rep_seq_y="[0 1 0 -1 0  ]"
  Repeating Sequence2 : simulink/Sources/Repeating Sequence  rep_seq_t=[0 0.00025 0.0005 0.00075 0.001]*(1/fr)*(1/fc)*(1/2)  rep_seq_y=[ 0 -1 0 1 0 ]
  Repeating Sequence5 : simulink/Sources/Repeating Sequence  rep_seq_t=[0 0.00025 0.0005 0.00075 0.001]*(1/fr)*(1/fc)*(1/2)  rep_seq_y=[1 0 -1 0 1]
  Repeating Sequence7 : simulink/Sources/Repeating Sequence  rep_seq_t=[0 0.00025 0.0005 0.00075 0.001]*(1/fr)*(1/fc)*(1/2)  rep_seq_y=[-1 0 1 0 -1]
  SW{1..8} (8 alike) : spsIGBTDiodeLib/IGBT//Diode  Ron=1e-3  Rs=1e5  Cs=inf  Measurements=on
  Sine Wave1 : Sin  Amplitude=Ma  Frequency=2*pi*fr  Phase=ph  SampleTime=0
  Sine Wave2 : Sin  Amplitude=Ma  Frequency=2*pi*fr  Phase=ph  SampleTime=0
  Va : PMIOPort  Tag=PMCPort  Side=Right
  N : PMIOPort  Tag=PMCPort  Port=2  Side=Right
  wires:
  Sine Wave2/1 -> Relational Operator4/1, Relational Operator6/1
  Repeating Sequence1/1 -> Relational Operator4/2
  Repeating Sequence2/1 -> Relational Operator6/2
  Relational Operator4/1 -> NOT/1, [S1]
  NOT/1 -> [S3]
  NOT1/1 -> [S4]
  Relational Operator6/1 -> [S2], NOT1/1
  Repeating Sequence7/1 -> Relational Operator7/2
  Repeating Sequence5/1 -> Relational Operator5/2
  Sine Wave1/1 -> Relational Operator7/1, Relational Operator5/1
  Relational Operator5/1 -> [S6], NOT3/1
  Relational Operator7/1 -> [S5], NOT2/1
  NOT2/1 -> [S7]
  NOT3/1 -> [S8]
  [S3] -> SW3/1
  [S4] -> SW4/1
  [S6] -> SW6/1
  [S5] -> SW5/1
  [S7] -> SW7/1
  [S8] -> SW8/1
  [S1] -> SW1/1
  [S2] -> SW2/1
  connections:
  Va/RConn1 -- SW2/RConn1 -- SW4/LConn1
  SW4/RConn1 -- 100V/LConn1 -- SW3/RConn1
  SW8/RConn1 -- 100V1/LConn1 -- SW7/RConn1
  SW6/RConn1 -- SW1/RConn1
  SW5/LConn1 -- 100V1/RConn1 -- SW6/LConn1
  N/RConn1 -- SW5/RConn1 -- SW7/LConn1
  100V/RConn1 -- SW1/LConn1 -- SW2/LConn1

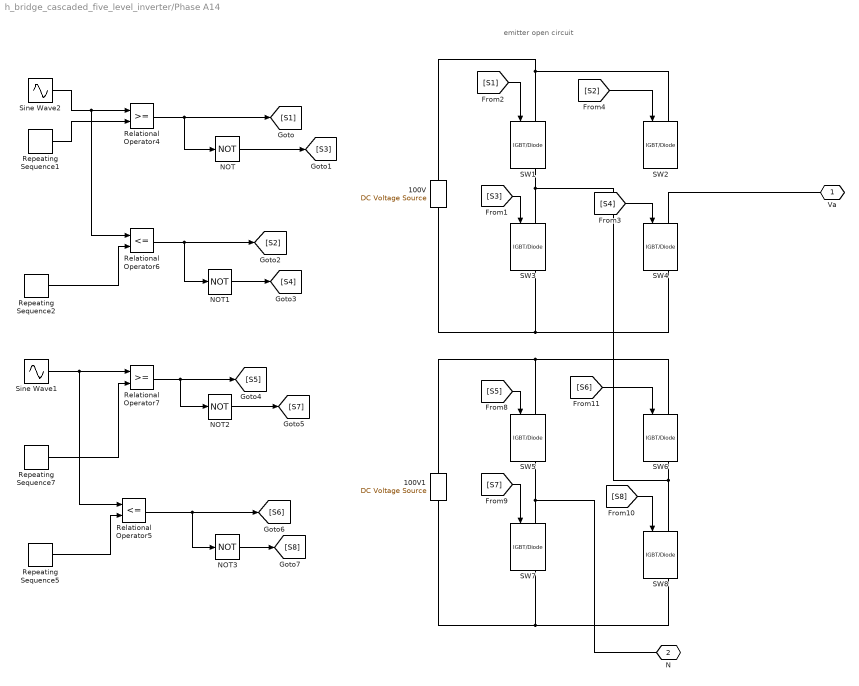
== system h_bridge_cascaded_five_level_inverter/Phase A14 ==
  note: emitter open circuit
  100V : spsDCVoltageSourceLib/DC Voltage Source  Amplitude=100  Measurements=None
  100V1 : spsDCVoltageSourceLib/DC Voltage Source  Amplitude=100  Measurements=None
  NOT{,1..3} (4 alike) : Logic  Operator=NOT  AllPortsSameDT=off  OutDataTypeStr=boolean
  Relational Operator4 : RelationalOperator  OutDataTypeStr=boolean  InputSameDT=off
  Relational Operator5 : RelationalOperator  Operator=<=  OutDataTypeStr=boolean  InputSameDT=off
  Relational Operator6 : RelationalOperator  Operator=<=  OutDataTypeStr=boolean  InputSameDT=off
  Relational Operator7 : RelationalOperator  OutDataTypeStr=boolean  InputSameDT=off
  Repeating Sequence1 : simulink/Sources/Repeating Sequence  rep_seq_t=[0 0.00025 0.0005 0.00075 0.001]*(1/fr)*(1/fc)*(1/2)  rep_seq_y="[0 1 0 -1 0  ]"
  Repeating Sequence2 : simulink/Sources/Repeating Sequence  rep_seq_t=[0 0.00025 0.0005 0.00075 0.001]*(1/fr)*(1/fc)*(1/2)  rep_seq_y=[ 0 -1 0 1 0 ]
  Repeating Sequence5 : simulink/Sources/Repeating Sequence  rep_seq_t=[0 0.00025 0.0005 0.00075 0.001]*(1/fr)*(1/fc)*(1/2)  rep_seq_y=[1 0 -1 0 1]
  Repeating Sequence7 : simulink/Sources/Repeating Sequence  rep_seq_t=[0 0.00025 0.0005 0.00075 0.001]*(1/fr)*(1/fc)*(1/2)  rep_seq_y=[-1 0 1 0 -1]
  SW{1..8} (8 alike) : spsIGBTDiodeLib/IGBT//Diode  Ron=1e-3  Rs=1e5  Cs=inf  Measurements=on
  Sine Wave1 : Sin  Amplitude=Ma  Frequency=2*pi*fr  Phase=ph  SampleTime=0
  Sine Wave2 : Sin  Amplitude=Ma  Frequency=2*pi*fr  Phase=ph  SampleTime=0
  Va : PMIOPort  Tag=PMCPort  Side=Right
  N : PMIOPort  Tag=PMCPort  Port=2  Side=Right
  wires:
  Sine Wave2/1 -> Relational Operator4/1, Relational Operator6/1
  Repeating Sequence1/1 -> Relational Operator4/2
  Repeating Sequence2/1 -> Relational Operator6/2
  Relational Operator4/1 -> NOT/1, [S1]
  NOT/1 -> [S3]
  NOT1/1 -> [S4]
  Relational Operator6/1 -> [S2], NOT1/1
  Repeating Sequence7/1 -> Relational Operator7/2
  Repeating Sequence5/1 -> Relational Operator5/2
  Sine Wave1/1 -> Relational Operator7/1, Relational Operator5/1
  Relational Operator5/1 -> [S6], NOT3/1
  Relational Operator7/1 -> [S5], NOT2/1
  NOT2/1 -> [S7]
  NOT3/1 -> [S8]
  [S3] -> SW3/1
  [S4] -> SW4/1
  [S6] -> SW6/1
  [S5] -> SW5/1
  [S7] -> SW7/1
  [S8] -> SW8/1
  [S1] -> SW1/1
  [S2] -> SW2/1
  connections:
  Va/RConn1 -- SW4/LConn1
  SW4/RConn1 -- 100V/LConn1 -- SW3/RConn1
  SW8/RConn1 -- 100V1/LConn1 -- SW7/RConn1
  SW3/LConn1 -- SW1/RConn1 -- SW6/RConn1 -- SW8/LConn1
  SW5/LConn1 -- 100V1/RConn1 -- SW6/LConn1
  N/RConn1 -- SW5/RConn1 -- SW7/LConn1
  100V/RConn1 -- SW1/LConn1 -- SW2/LConn1

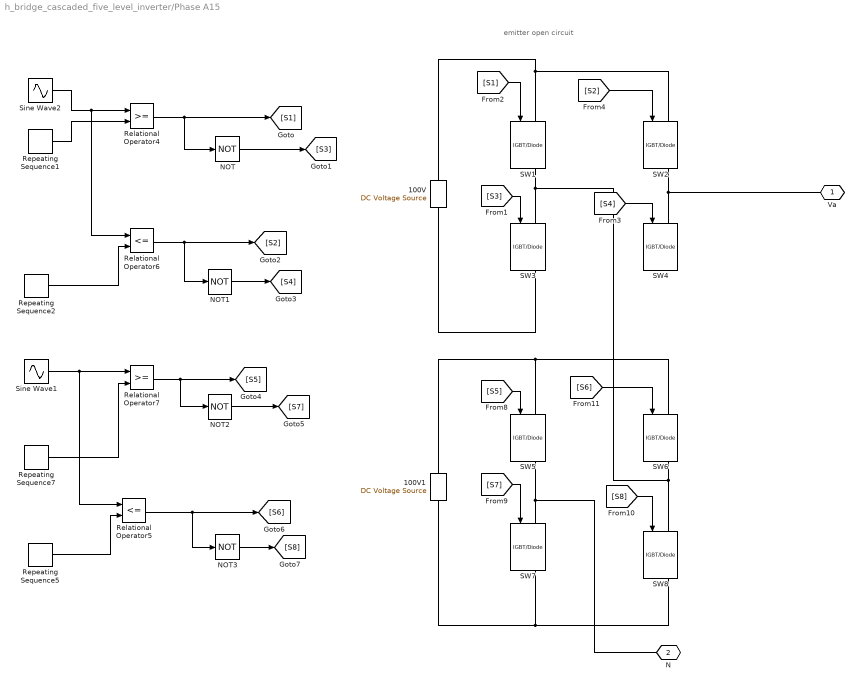
== system h_bridge_cascaded_five_level_inverter/Phase A15 ==
  note: emitter open circuit
  100V : spsDCVoltageSourceLib/DC Voltage Source  Amplitude=100  Measurements=None
  100V1 : spsDCVoltageSourceLib/DC Voltage Source  Amplitude=100  Measurements=None
  NOT{,1..3} (4 alike) : Logic  Operator=NOT  AllPortsSameDT=off  OutDataTypeStr=boolean
  Relational Operator4 : RelationalOperator  OutDataTypeStr=boolean  InputSameDT=off
  Relational Operator5 : RelationalOperator  Operator=<=  OutDataTypeStr=boolean  InputSameDT=off
  Relational Operator6 : RelationalOperator  Operator=<=  OutDataTypeStr=boolean  InputSameDT=off
  Relational Operator7 : RelationalOperator  OutDataTypeStr=boolean  InputSameDT=off
  Repeating Sequence1 : simulink/Sources/Repeating Sequence  rep_seq_t=[0 0.00025 0.0005 0.00075 0.001]*(1/fr)*(1/fc)*(1/2)  rep_seq_y="[0 1 0 -1 0  ]"
  Repeating Sequence2 : simulink/Sources/Repeating Sequence  rep_seq_t=[0 0.00025 0.0005 0.00075 0.001]*(1/fr)*(1/fc)*(1/2)  rep_seq_y=[ 0 -1 0 1 0 ]
  Repeating Sequence5 : simulink/Sources/Repeating Sequence  rep_seq_t=[0 0.00025 0.0005 0.00075 0.001]*(1/fr)*(1/fc)*(1/2)  rep_seq_y=[1 0 -1 0 1]
  Repeating Sequence7 : simulink/Sources/Repeating Sequence  rep_seq_t=[0 0.00025 0.0005 0.00075 0.001]*(1/fr)*(1/fc)*(1/2)  rep_seq_y=[-1 0 1 0 -1]
  SW{1..8} (8 alike) : spsIGBTDiodeLib/IGBT//Diode  Ron=1e-3  Rs=1e5  Cs=inf  Measurements=on
  Sine Wave1 : Sin  Amplitude=Ma  Frequency=2*pi*fr  Phase=ph  SampleTime=0
  Sine Wave2 : Sin  Amplitude=Ma  Frequency=2*pi*fr  Phase=ph  SampleTime=0
  Va : PMIOPort  Tag=PMCPort  Side=Right
  N : PMIOPort  Tag=PMCPort  Port=2  Side=Right
  wires:
  Sine Wave2/1 -> Relational Operator4/1, Relational Operator6/1
  Repeating Sequence1/1 -> Relational Operator4/2
  Repeating Sequence2/1 -> Relational Operator6/2
  Relational Operator4/1 -> NOT/1, [S1]
  NOT/1 -> [S3]
  NOT1/1 -> [S4]
  Relational Operator6/1 -> [S2], NOT1/1
  Repeating Sequence7/1 -> Relational Operator7/2
  Repeating Sequence5/1 -> Relational Operator5/2
  Sine Wave1/1 -> Relational Operator7/1, Relational Operator5/1
  Relational Operator5/1 -> [S6], NOT3/1
  Relational Operator7/1 -> [S5], NOT2/1
  NOT2/1 -> [S7]
  NOT3/1 -> [S8]
  [S3] -> SW3/1
  [S4] -> SW4/1
  [S6] -> SW6/1
  [S5] -> SW5/1
  [S7] -> SW7/1
  [S8] -> SW8/1
  [S1] -> SW1/1
  [S2] -> SW2/1
  connections:
  Va/RConn1 -- SW2/RConn1 -- SW4/LConn1
  SW3/RConn1 -- 100V/LConn1
  SW8/RConn1 -- 100V1/LConn1 -- SW7/RConn1
  SW3/LConn1 -- SW1/RConn1 -- SW8/LConn1 -- SW6/RConn1
  SW5/LConn1 -- 100V1/RConn1 -- SW6/LConn1
  N/RConn1 -- SW5/RConn1 -- SW7/LConn1
  100V/RConn1 -- SW1/LConn1 -- SW2/LConn1
